simulink library "gpkfPathOptWithRGPinnerLoop_cl"  (R2020a)
settings: Solver=VariableStepAuto  StartTime=0.0  StopTime=10.0  RelTol=1e-3
undefined symbols (not defined in the file or in its folder): HILVLCONTROLLER, hiLvlCtrl, initializeBussesFromBlock
libraries: calculate_vector_magnitude x3, simulink x1, optimizePathShapeRGP_ul x1, calc_Lap_Average x1, dspsigops x1, calcKalmanEstimate_ul x1, optimizeTrajectory_ul x1
settings Model: Creator=Ayaz  LastModifiedBy=Ayaz

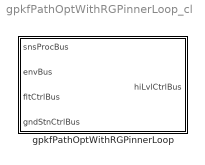
== system gpkfPathOptWithRGPinnerLoop_cl ==
  gpkfPathOptWithRGPinnerLoop : Subsystem  LoadFcn=initializeBussesFromBlock(gcb)  InitFcn=initializeBussesFromBlock(gcb)  StartFcn=initializeBussesFromBlock(gcb)  VariantControl=strcmpi(HILVLCONTROLLER,'gpkfPathOptWithRGPinnerLoop')  mask{hiLvlCtrl=hiLvlCtrl}
      mask prompts: hiLvlCtrl "Hi-level controller object"
      mask TypeOptions hiLvlCtrl: gpkfPathOpt/hiLvlCtrl

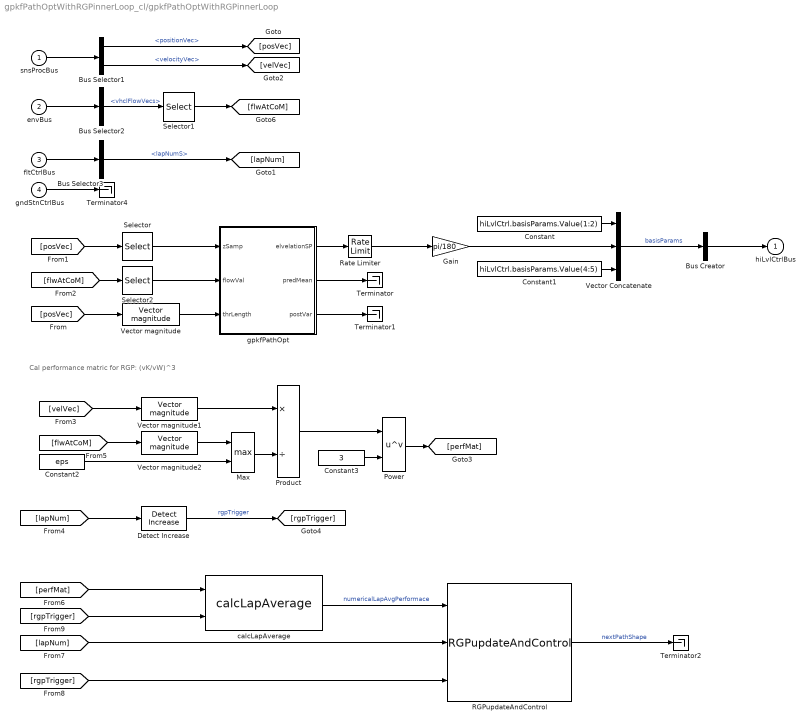
== system gpkfPathOptWithRGPinnerLoop_cl/gpkfPathOptWithRGPinnerLoop ==
  note: Cal performance matric for RGP: (vK/vW)^3
  snsProcBus : Inport
  envBus : Inport  Port=2
  fltCtrlBus : Inport  Port=3
  gndStnCtrlBus : Inport  Port=4
  Bus Creator : BusCreator  Inputs=1  OutDataTypeStr=Bus: hiLvlCtrlBus
  Bus Selector1 : BusSelector  OutputSignals=positionVec,velocityVec
  Bus Selector2 : BusSelector  OutputSignals=vhclFlowVecs
  Bus Selector3 : BusSelector  OutputSignals=lapNumS
  Constant : Constant  Value=hiLvlCtrl.basisParams.Value(1:2)
  Constant1 : Constant  Value=hiLvlCtrl.basisParams.Value(4:5)
  Constant2 : Constant  Value=eps
  Constant3 : Constant  Value=3
  Detect Increase : simulink/Logic and Bit Operations/Detect Increase  vinit=0.0  OutDataTypeStr=boolean
  Gain : Gain  Gain=pi/180
  Max : MinMax  Function=max  Inputs=2
  Power : Math  Operator=pow  SaturateOnIntegerOverflow=on
  Product : Product  Inputs=*/
  RGPupdateAndControl : optimizePathShapeRGP_ul/RGPupdateAndControl  hiLvlCtrl=hiLvlCtrl
  Rate Limiter : RateLimiter  RisingSlewLimit=hiLvlCtrl.rateLimit  FallingSlewLimit=-hiLvlCtrl.rateLimit  SampleTimeMode=inherited
  Selector : Selector  NumberOfDimensions=2  InputPortWidth=3  IndexOptions=Index vector (dialog),Index vector (dialog)  Indices=3,1  OutputSizes=1,1
  Selector1 : Selector  NumberOfDimensions=2  InputPortWidth=3  IndexOptions=Select all,Index vector (dialog)  Indices=[1 3],5  OutputSizes=1,1
  Selector2 : Selector  NumberOfDimensions=2  InputPortWidth=3  IndexOptions=Index vector (dialog),Index vector (dialog)  Indices=1,1  OutputSizes=1,1
  Terminator{,1..2,4} (4 alike) : Terminator
  Vector Concatenate : Concatenate  NumInputs=3
  Vector magnitude : calculate_vector_magnitude/Vector magnitude  SystemSampleTime=-1  Latency=0  AutoFrameSizeCalculation=off
  Vector magnitude1 : calculate_vector_magnitude/Vector magnitude  SystemSampleTime=-1  Latency=0  AutoFrameSizeCalculation=off
  Vector magnitude2 : calculate_vector_magnitude/Vector magnitude  SystemSampleTime=-1  Latency=0  AutoFrameSizeCalculation=off
  calcLapAverage : calc_Lap_Average/calcLapAverage  SystemSampleTime=-1  Latency=0  AutoFrameSizeCalculation=off
  gpkfPathOpt : Subsystem  mask{hiLvlCtrl=hiLvlCtrl}
      mask prompts: hiLvlCtrl "Hi-level controller object"
      mask TypeOptions hiLvlCtrl: calcKalmanEstimate/hiLvlCtrl | optimizeMeanElevation/hiLvlCtrl
  hiLvlCtrlBus : Outport
  wires:
  Bus Selector1/2 -> [velVec]  "<velocityVec>"
  Bus Selector3/1 -> [lapNum]  "<lapNumS>"
  fltCtrlBus/1 -> Bus Selector3/1
  Selector1/1 -> [flwAtCoM]
  [flwAtCoM] -> Selector2/1
  Bus Selector2/1 -> Selector1/1  "<vhclFlowVecs>"
  Selector2/1 -> gpkfPathOpt/2(flowVal)
  Constant1/1 -> Vector Concatenate/3
  Rate Limiter/1 -> Gain/1
  Constant/1 -> Vector Concatenate/1
  Vector Concatenate/1 -> Bus Creator/1  "basisParams"
  Gain/1 -> Vector Concatenate/2
  [posVec] -> Selector/1
  Selector/1 -> gpkfPathOpt/1(zSamp)
  gpkfPathOpt/1(elvelationSP) -> Rate Limiter/1
  Vector magnitude/1 -> gpkfPathOpt/3(thrLength)
  [posVec] -> Vector magnitude/1
  gpkfPathOpt/2(predMean) -> Terminator/1
  snsProcBus/1 -> Bus Selector1/1
  Bus Selector1/1 -> [posVec]  "<positionVec>"
  envBus/1 -> Bus Selector2/1
  Bus Creator/1 -> hiLvlCtrlBus/1
  gpkfPathOpt/3(postVar) -> Terminator1/1
  gndStnCtrlBus/1 -> Terminator4/1
  [perfMat] -> calcLapAverage/1
  calcLapAverage/1 -> RGPupdateAndControl/1  "numericalLapAvgPerformace"
  [velVec] -> Vector magnitude1/1
  [flwAtCoM] -> Vector magnitude2/1
  Vector magnitude1/1 -> Product/1
  Vector magnitude2/1 -> Max/1
  Max/1 -> Product/2
  Constant2/1 -> Max/2
  Product/1 -> Power/1
  Constant3/1 -> Power/2
  Power/1 -> [perfMat]
  [lapNum] -> RGPupdateAndControl/2
  Detect Increase/1 -> [rgpTrigger]  "rgpTrigger"
  [lapNum] -> Detect Increase/1
  [rgpTrigger] -> RGPupdateAndControl/3
  [rgpTrigger] -> calcLapAverage/2
  RGPupdateAndControl/1 -> Terminator2/1  "nextPathShape"

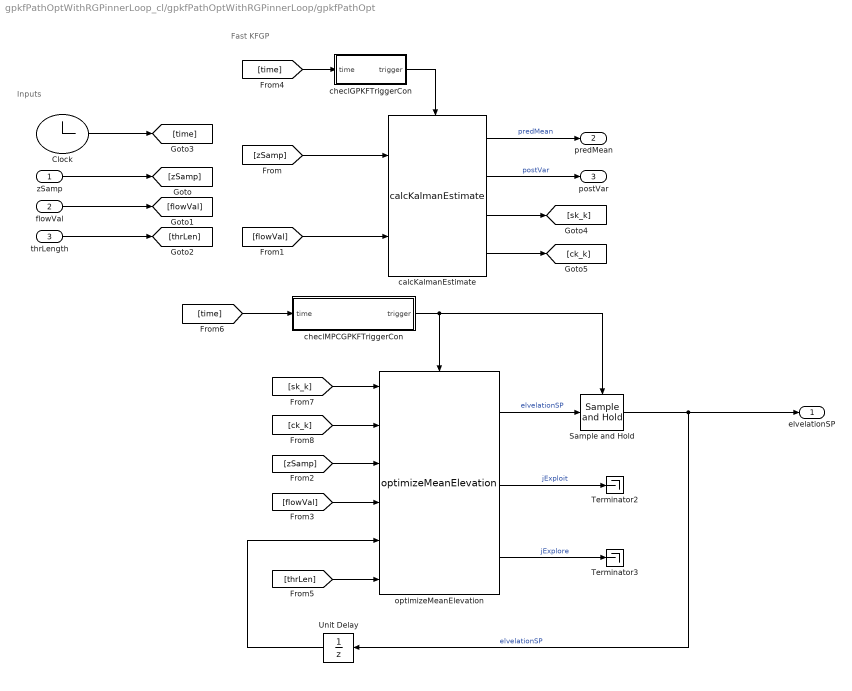
== system gpkfPathOptWithRGPinnerLoop_cl/gpkfPathOptWithRGPinnerLoop/gpkfPathOpt ==
  note: Fast KFGP
  note: Inputs
  zSamp : Inport
  flowVal : Inport  Port=2
  thrLength : Inport  Port=3
  Clock : Clock
      settings: Decimation=2
  Sample and Hold : dspsigops/Sample and Hold  trig=Rising edge  initCond=hiLvlCtrl.initVals  latchinput=off
  Terminator2 : Terminator
  Terminator3 : Terminator
  Unit Delay : UnitDelay  InitialCondition=hiLvlCtrl.initVals  SampleTime=-1  HasFrameUpgradeWarning=on
  calcKalmanEstimate : calcKalmanEstimate_ul/calcKalmanEstimate  hiLvlCtrl=hiLvlCtrl
  checlGPKFTriggerCon : Subsystem
  checlMPCGPKFTriggerCon : Subsystem
  optimizeMeanElevation : optimizeTrajectory_ul/optimizeMeanElevation  hiLvlCtrl=hiLvlCtrl
  elvelationSP : Outport
  predMean : Outport  Port=2
  postVar : Outport  Port=3
  wires:
  calcKalmanEstimate/3 -> [sk_k]
  calcKalmanEstimate/4 -> [ck_k]
  flowVal/1 -> [flowVal]
  zSamp/1 -> [zSamp]
  [zSamp] -> calcKalmanEstimate/1
  [flowVal] -> calcKalmanEstimate/2
  [zSamp] -> optimizeMeanElevation/3
  [flowVal] -> optimizeMeanElevation/4
  thrLength/1 -> [thrLen]
  Unit Delay/1 -> optimizeMeanElevation/5
  [thrLen] -> optimizeMeanElevation/6
  calcKalmanEstimate/1 -> predMean/1  "predMean"
  calcKalmanEstimate/2 -> postVar/1  "postVar"
  optimizeMeanElevation/2 -> Terminator2/1  "jExploit"
  optimizeMeanElevation/3 -> Terminator3/1  "jExplore"
  Sample and Hold/1 -> elvelationSP/1, Unit Delay/1  "elvelationSP"
  Clock/1 -> [time]
  [time] -> checlGPKFTriggerCon/1(time)
  checlGPKFTriggerCon/1(trigger) -> calcKalmanEstimate/Enable
  [time] -> checlMPCGPKFTriggerCon/1(time)
  checlMPCGPKFTriggerCon/1(trigger) -> Sample and Hold/Trigger, optimizeMeanElevation/Enable
  optimizeMeanElevation/1 -> Sample and Hold/1  "elvelationSP"
  [sk_k] -> optimizeMeanElevation/1
  [ck_k] -> optimizeMeanElevation/2

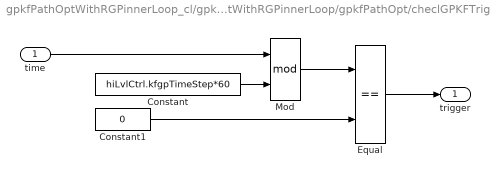
== system gpkfPathOptWithRGPinnerLoop_cl/gpkfPathOptWithRGPinnerLoop/gpkfPathOpt/checlGPKFTriggerCon ==
  time : Inport
  Constant : Constant  Value=hiLvlCtrl.kfgpTimeStep*60
  Constant1 : Constant  Value=0
  Equal : RelationalOperator  Operator===  OutDataTypeStr=boolean  RndMeth=Simplest
  Mod : Math  Operator=mod  SaturateOnIntegerOverflow=on
  trigger : Outport
  wires:
  Mod/1 -> Equal/1
  Constant1/1 -> Equal/2
  time/1 -> Mod/1
  Equal/1 -> trigger/1
  Constant/1 -> Mod/2

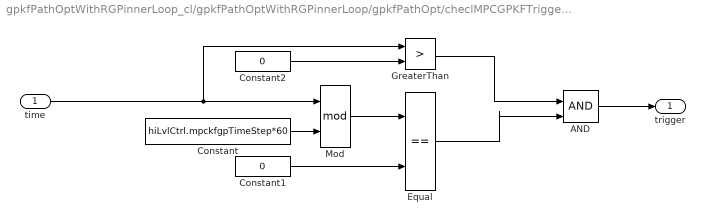
== system gpkfPathOptWithRGPinnerLoop_cl/gpkfPathOptWithRGPinnerLoop/gpkfPathOpt/checlMPCGPKFTriggerCon ==
  time : Inport
  AND : Logic  IconShape=distinctive  AllPortsSameDT=off  OutDataTypeStr=boolean
  Constant : Constant  Value=hiLvlCtrl.mpckfgpTimeStep*60
  Constant1 : Constant  Value=0
  Constant2 : Constant  Value=0
  Equal : RelationalOperator  Operator===  OutDataTypeStr=boolean  RndMeth=Simplest
  GreaterThan : RelationalOperator  Operator=>  OutDataTypeStr=boolean  RndMeth=Simplest
  Mod : Math  Operator=mod  SaturateOnIntegerOverflow=on
  trigger : Outport
  wires:
  Mod/1 -> Equal/1
  Constant/1 -> Mod/2
  time/1 -> GreaterThan/1, Mod/1
  Constant1/1 -> Equal/2
  Constant2/1 -> GreaterThan/2
  Equal/1 -> AND/2
  GreaterThan/1 -> AND/1
  AND/1 -> trigger/1
